simulink model "path_following_controller"  (R2020b)
settings: Solver=VariableStepAuto  StartTime=0.0  StopTime=10.0  RelTol=1e-3
values from neighbouring files (symbols this model uses):
  k_phi = sqrt(4.*k_rho) + 0.2    [main.m]
  k_rho = 0.7    [main.m]
  v_o = 1.2    [main.m]
libraries: roblocks x1
settings Model: Creator=Raj  LastModifiedBy=Raj

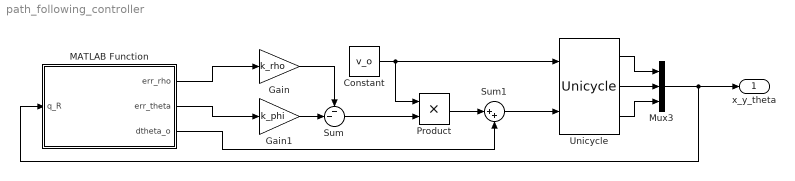
== system path_following_controller ==
  Constant : Constant  Value=v_o  VectorParams1D=off  SampleTime=0.02
  Gain : Gain  Gain=k_rho
  Gain1 : Gain  Gain=k_phi
  MATLAB Function : MATLAB Function  TreatAsAtomicUnit=on
  Mux3 : Mux  Inputs=3
  Product : Product
  Sum : Sum  Inputs=--|
  Sum1 : Sum  Inputs=|++
  Unicycle : roblocks/Vehicles/Unicycle  alim=acc  vlim=v_o  wlim=turn_rt_lim  x0=x0  a=frame_shift
  x_y_theta : Outport  VectorParamsAs1DForOutWhenUnconnected=off
  wires:
  MATLAB Function/3(dtheta_o) -> Sum1/2
  Constant/1 -> Unicycle/1, Product/1
  Sum/1 -> Product/2
  Sum1/1 -> Unicycle/2
  Unicycle/3 -> Mux3/3
  Gain1/1 -> Sum/2
  Product/1 -> Sum1/1
  MATLAB Function/1(err_rho) -> Gain/1
  Unicycle/1 -> Mux3/1
  MATLAB Function/2(err_theta) -> Gain1/1
  Unicycle/2 -> Mux3/2
  Gain/1 -> Sum/1
  Mux3/1 -> x_y_theta/1, MATLAB Function/1(q_R)

== matlab function path_following_controller/MATLAB Function ==
  settings: updateMethod=DISCRETE
  data: err_rho output; q_R input; err_theta output; dtheta_o output; rho_o parameter
function [err_rho, err_theta, dtheta_o] = path_dynamics(q_R, rho_o)
    [err_rho, err_theta, dtheta_o] = path_dynamics(q_R, rho_o);
end
